simulink model "lab3controller"  (R2024a)
settings: Solver=ode45  StartTime=0.0  StopTime=1  MaxStep=0.001  RelTol=1e-3
values from neighbouring files (symbols this model uses):
  K_d = 0.031    [lab3.m]
  K_p = 19.4    [lab3.m]
  K_r = 1 + 3/5/K_p    (= 1.03092783505)    [lab3.m]
  t_d = 0    [lab3.m]
  w_r = 1    [lab3.m]
settings Model: Creator=rar4  LastModifiedBy=xinchen
settings RTWCC: GPUComputeCapability=3.5

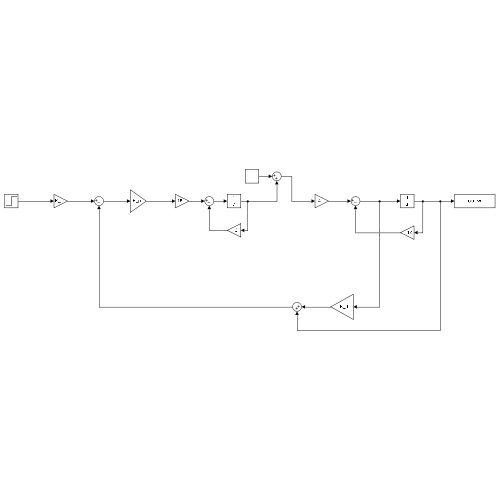
[thumbnail: Simulink's stored preview of the top-level diagram]
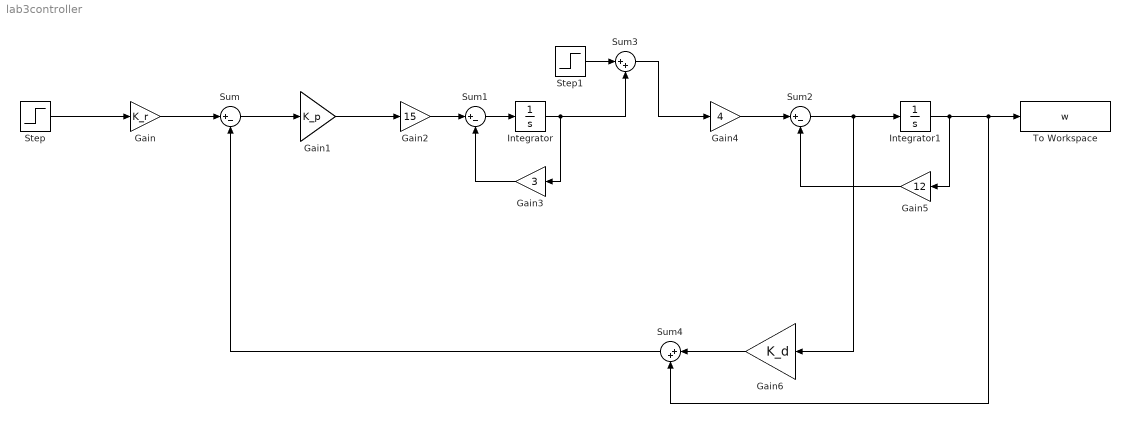
== system lab3controller ==
  Gain : Gain  Gain=K_r
  Gain1 : Gain  Gain=K_p
  Gain2 : Gain  Gain=15
  Gain3 : Gain  Gain=3
  Gain4 : Gain  Gain=4
  Gain5 : Gain  Gain=12
  Gain6 : Gain  Gain=K_d
  Integrator : Integrator
  Integrator1 : Integrator
  Step : Step  Time=0  Before=w_r  After=w_r  SampleTime=0
  Step1 : Step  Time=0  Before=t_d  After=t_d  SampleTime=0
  Sum : Sum  Inputs=|+-
  Sum1 : Sum  Inputs=|+-
  Sum2 : Sum  Inputs=|+-
  Sum3 : Sum  Inputs=|++
  Sum4 : Sum  Inputs=|++
  To Workspace : ToWorkspace  VariableName=w  SampleTime=-1
  wires:
  Step/1 -> Gain/1
  Gain/1 -> Sum/1
  Sum/1 -> Gain1/1
  Gain1/1 -> Gain2/1
  Gain2/1 -> Sum1/1
  Sum1/1 -> Integrator/1
  Integrator/1 -> Sum3/2, Gain3/1
  Gain3/1 -> Sum1/2
  Step1/1 -> Sum3/1
  Sum3/1 -> Gain4/1
  Gain4/1 -> Sum2/1
  Sum2/1 -> Integrator1/1, Gain6/1
  Gain5/1 -> Sum2/2
  Gain6/1 -> Sum4/1
  Integrator1/1 -> Sum4/2, To Workspace/1, Gain5/1
  Sum4/1 -> Sum/2
